simulink model "gimbal_cmd_unit_test"  (R2015b)
settings: Solver=FixedStepDiscrete  StartTime=0.0  StopTime=200  FixedStep=0.1  RelTol=1e-3
values from neighbouring files (symbols this model uses):
  Bm = 0.1    [gimbal_cmd_test.m]    (also in resolve_gimbal_angle_from_true_actuator_length.m)
  Jm = 0.01    [gimbal_cmd_test.m]    (also in resolve_gimbal_angle_from_true_actuator_length.m)
  Ke = 0.01    [gimbal_cmd_test.m]    (also in resolve_gimbal_angle_from_true_actuator_length.m)
  Kl = 500    [gimbal_cmd_test.m]    (also in resolve_gimbal_angle_from_true_actuator_length.m = 5000)
  Kt = 0.01    [gimbal_cmd_test.m]    (also in resolve_gimbal_angle_from_true_actuator_length.m)
  Lm = 0.5    [gimbal_cmd_test.m]    (also in resolve_gimbal_angle_from_true_actuator_length.m)
  mass = 50    [gimbal_cmd_test.m]
  nb = 2e-2/(2*pi)    (= 0.00318309886184)    [gimbal_cmd_test.m]    (also in resolve_gimbal_angle_from_true_actuator_length.m)
  Rm = 1    [gimbal_cmd_test.m]    (also in resolve_gimbal_angle_from_true_actuator_length.m)
  rot_err_x_rad = -1*pi/180    (= -0.0174532925199)    [gimbal_cmd_test.m]
  rot_err_y_rad = 0.0    (= 0)    [gimbal_cmd_test.m]
  rot_err_z_rad = 1*pi/180    (= 0.0174532925199)    [gimbal_cmd_test.m]
  w_err_x_rad = 0.0    (= 0)    [gimbal_cmd_test.m]
  w_err_y_rad = 0.0    (= 0)    [gimbal_cmd_test.m]
  w_err_z_rad = 0.0    (= 0)    [gimbal_cmd_test.m]
undefined symbols (not defined in the file or in its folder): DiscIntNeverNeededParam, tpl_x_gimbal_actuator_to_angle
libraries: util_quat_lib x2, simulink x1, simulink_extras x1, csc_vac_gimbal_steering_vernier_roll_acs_ctrl_lib_diag x1
settings Model: Creator=jimkaidy  LastModifiedBy=jimkaidy

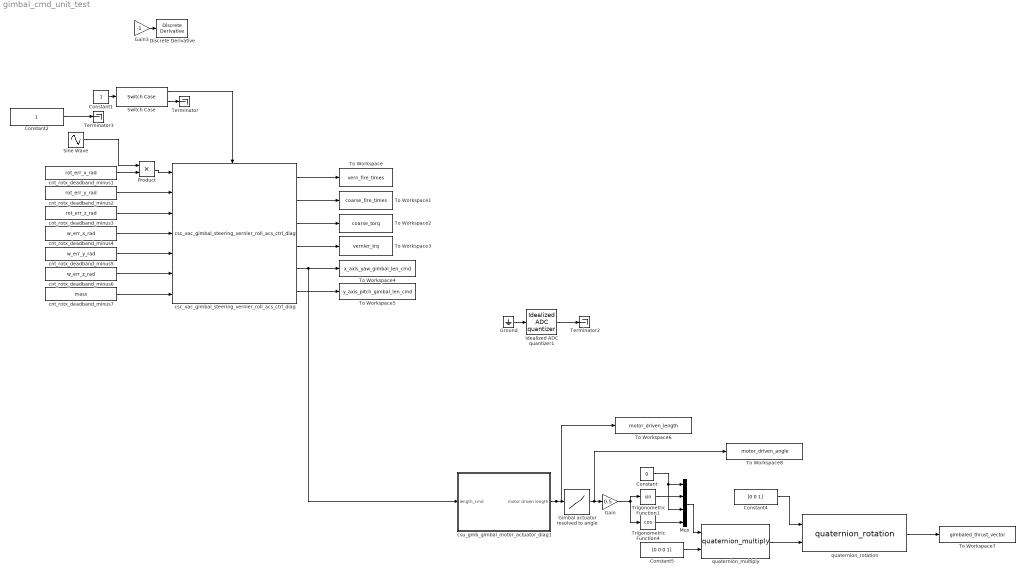
== system gimbal_cmd_unit_test ==
  Constant : Constant  Value=0
  Constant1 : Constant  OutDataTypeStr=uint8
  Constant2 : Constant  OutDataTypeStr=uint8
  Constant4 : Constant  Value=[0 0 1]
  Constant5 : Constant  Value=[0 0 0 1]
  Discrete Derivative : simulink/Discrete/Discrete Derivative  gainval=1.0  ICPrevScaledInput=0.0  InputProcessing=Inherited  OutMin=[]  OutMax=[]  OutDataType=fixdt(1, 16)  OutScaling=2^-10  DoSatur=off
  Gain : Gain  Gain=0.5
  Gain3 : Gain  Gain=-1
  Gimbal actuator resolved to angle : Lookup  InputValues=tpl_x_gimbal_actuator_to_angle(:,1)  Table=tpl_x_gimbal_actuator_to_angle(:,2)  LookUpMeth=Interpolation-Use End Values
  Ground : Ground
  Idealized ADC quantizer1 : simulink_extras/Additional Discrete/Idealized ADC quantizer  NumberOfConverterBits=12  Vmin=-10  Vmax=10  OutputDataType=int16  OutputNegativeValues=off
  Mux : Mux
  Product : Product
  Sine Wave : Sin  Frequency=10*pi/180  SampleTime=0.1
  Switch Case : SwitchCase
  Terminator : Terminator
  Terminator2 : Terminator
  Terminator3 : Terminator
  To Workspace : ToWorkspace  VariableName=vern_fire_times  SaveFormat=Timeseries  SampleTime=-1
  To Workspace1 : ToWorkspace  VariableName=coarse_fire_times  SaveFormat=Timeseries  SampleTime=-1
  To Workspace2 : ToWorkspace  VariableName=coarse_torq  SaveFormat=Timeseries  SampleTime=-1
  To Workspace3 : ToWorkspace  VariableName=vernier_trq  SaveFormat=Timeseries  SampleTime=-1
  To Workspace4 : ToWorkspace  VariableName=x_axis_yaw_gimbal_len_cmd  SaveFormat=Timeseries  SampleTime=-1
  To Workspace5 : ToWorkspace  VariableName=y_axis_pitch_gimbal_len_cmd  SaveFormat=Timeseries  SampleTime=-1
  To Workspace6 : ToWorkspace  VariableName=motor_driven_length  SaveFormat=Timeseries  SampleTime=-1
  To Workspace7 : ToWorkspace  VariableName=gimbaled_thrust_vector  SaveFormat=Timeseries  SampleTime=-1
  To Workspace8 : ToWorkspace  VariableName=motor_driven_angle  SaveFormat=Timeseries  SampleTime=-1
  Trigonometric Function1 : Trigonometry
  Trigonometric Function4 : Trigonometry  Operator=cos
  cnt_rotx_deadband_minus1 : Constant  Value=rot_err_x_rad
  cnt_rotx_deadband_minus2 : Constant  Value=rot_err_y_rad
  cnt_rotx_deadband_minus3 : Constant  Value=rot_err_z_rad
  cnt_rotx_deadband_minus4 : Constant  Value=w_err_x_rad
  cnt_rotx_deadband_minus5 : Constant  Value=w_err_y_rad
  cnt_rotx_deadband_minus6 : Constant  Value=w_err_z_rad
  cnt_rotx_deadband_minus7 : Constant  Value=mass
  csc_vac_gimbal_steering_vernier_roll_acs_ctrl_diag : csc_vac_gimbal_steering_vernier_roll_acs_ctrl_lib_diag/csc_vac_gimbal_steering_vernier_roll_acs_ctrl_diag
  csu_gmb_gimbal_motor_actuator_diag1 : Subsystem
  quaternion_multiply : util_quat_lib/quaternion_multiply  SystemSampleTime=-1
  quaternion_rotation : util_quat_lib/quaternion_rotation  SystemSampleTime=-1
  wires:
  cnt_rotx_deadband_minus7/1 -> csc_vac_gimbal_steering_vernier_roll_acs_ctrl_diag/7
  cnt_rotx_deadband_minus2/1 -> csc_vac_gimbal_steering_vernier_roll_acs_ctrl_diag/2
  cnt_rotx_deadband_minus3/1 -> csc_vac_gimbal_steering_vernier_roll_acs_ctrl_diag/3
  cnt_rotx_deadband_minus5/1 -> csc_vac_gimbal_steering_vernier_roll_acs_ctrl_diag/5
  cnt_rotx_deadband_minus6/1 -> csc_vac_gimbal_steering_vernier_roll_acs_ctrl_diag/6
  csc_vac_gimbal_steering_vernier_roll_acs_ctrl_diag/1 -> To Workspace/1
  csc_vac_gimbal_steering_vernier_roll_acs_ctrl_diag/2 -> To Workspace1/1
  csc_vac_gimbal_steering_vernier_roll_acs_ctrl_diag/3 -> To Workspace2/1
  csc_vac_gimbal_steering_vernier_roll_acs_ctrl_diag/4 -> To Workspace3/1
  csc_vac_gimbal_steering_vernier_roll_acs_ctrl_diag/6 -> To Workspace5/1
  Constant1/1 -> Switch Case/1
  Switch Case/1 -> csc_vac_gimbal_steering_vernier_roll_acs_ctrl_diag/Action
  Switch Case/2 -> Terminator/1
  Product/1 -> csc_vac_gimbal_steering_vernier_roll_acs_ctrl_diag/1
  cnt_rotx_deadband_minus1/1 -> Product/2
  Sine Wave/1 -> Product/1
  cnt_rotx_deadband_minus4/1 -> csc_vac_gimbal_steering_vernier_roll_acs_ctrl_diag/4
  Idealized ADC quantizer1/1 -> Terminator2/1
  Ground/1 -> Idealized ADC quantizer1/1
  csu_gmb_gimbal_motor_actuator_diag1/1(motor driven length) -> To Workspace6/1, Gimbal actuator resolved to angle/1
  Gimbal actuator resolved to angle/1 -> To Workspace8/1, Gain/1
  Gain/1 -> Trigonometric Function4/1, Trigonometric Function1/1
  Trigonometric Function4/1 -> Mux/4
  Trigonometric Function1/1 -> Mux/2
  Constant/1 -> Mux/3, Mux/1
  Mux/1 -> quaternion_multiply/1
  quaternion_multiply/1 -> quaternion_rotation/2
  Constant4/1 -> quaternion_rotation/1
  quaternion_rotation/1 -> To Workspace7/1
  csc_vac_gimbal_steering_vernier_roll_acs_ctrl_diag/5 -> csu_gmb_gimbal_motor_actuator_diag1/1(length_cmd), To Workspace4/1
  Constant5/1 -> quaternion_multiply/2
  Gain3/1 -> Discrete Derivative/1
  Constant2/1 -> Terminator3/1

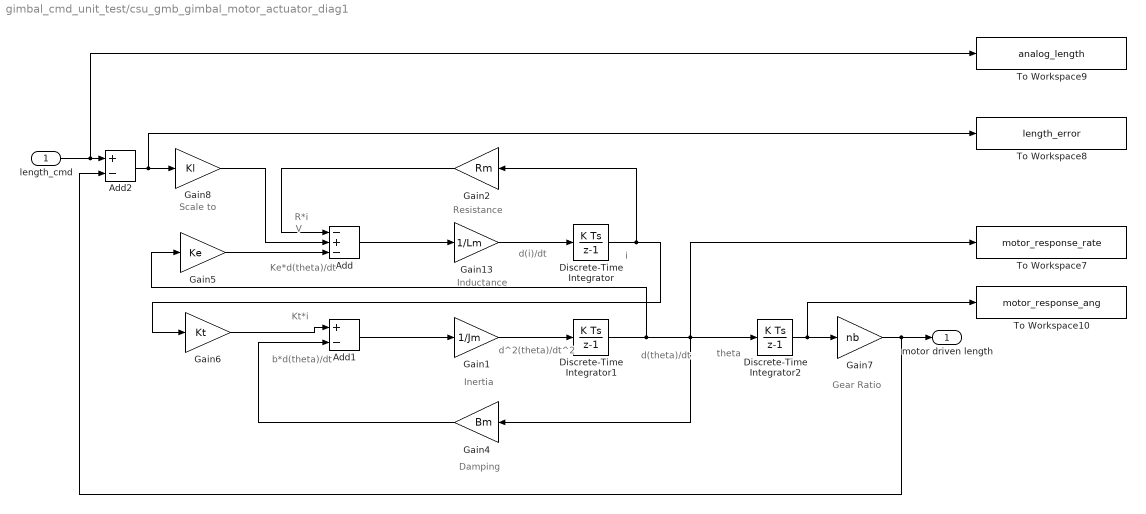
== system gimbal_cmd_unit_test/csu_gmb_gimbal_motor_actuator_diag1 ==
  note: Scale to
  note: theta
  note: d^2(theta)/dt^2
  note: b*d(theta)/dt
  note: Kt*i
  note: d(theta)/dt
  note: Ke*d(theta)/dt
  note: V
  note: R*i
  note: i
  note: d(i)/dt
  note: Gear Ratio
  note: Resistance
  note: Damping
  note: Inertia
  note: Inductance
  length_cmd : Inport
  Add : Sum  Inputs=-+-
  Add1 : Sum  Inputs=+-
  Add2 : Sum  Inputs=+-
  Discrete-Time Integrator : DiscreteIntegrator  InitialConditionSetting=State (most efficient)  SampleTime=-1  ICPrevOutput=DiscIntNeverNeededParam  ICPrevScaledInput=DiscIntNeverNeededParam
  Discrete-Time Integrator1 : DiscreteIntegrator  InitialConditionSetting=State (most efficient)  SampleTime=-1  ICPrevOutput=DiscIntNeverNeededParam  ICPrevScaledInput=DiscIntNeverNeededParam
  Discrete-Time Integrator2 : DiscreteIntegrator  InitialConditionSetting=State (most efficient)  SampleTime=-1  ICPrevOutput=DiscIntNeverNeededParam  ICPrevScaledInput=DiscIntNeverNeededParam
  Gain1 : Gain  Gain=1/Jm
  Gain13 : Gain  Gain=1/Lm
  Gain2 : Gain  Gain=Rm
  Gain4 : Gain  Gain=Bm
  Gain5 : Gain  Gain=Ke
  Gain6 : Gain  Gain=Kt
  Gain7 : Gain  Gain=nb
  Gain8 : Gain  Gain=Kl
  To Workspace10 : ToWorkspace  VariableName=motor_response_ang  SaveFormat=Timeseries  SampleTime=-1
  To Workspace7 : ToWorkspace  VariableName=motor_response_rate  SaveFormat=Timeseries  SampleTime=-1
  To Workspace8 : ToWorkspace  VariableName=length_error  SaveFormat=Timeseries  SampleTime=-1
  To Workspace9 : ToWorkspace  VariableName=analog_length  SaveFormat=Timeseries  SampleTime=-1
  motor driven length : Outport
  wires:
  length_cmd/1 -> To Workspace9/1, Add2/1
  Gain13/1 -> Discrete-Time Integrator/1
  Gain1/1 -> Discrete-Time Integrator1/1
  Gain5/1 -> Add/3
  Gain4/1 -> Add1/2
  Gain2/1 -> Add/1
  Gain6/1 -> Add1/1
  Discrete-Time Integrator/1 -> Gain2/1, Gain6/1
  Gain8/1 -> Add/2
  Add/1 -> Gain13/1
  Add1/1 -> Gain1/1
  Discrete-Time Integrator1/1 -> Gain5/1, To Workspace7/1, Gain4/1, Discrete-Time Integrator2/1
  Add2/1 -> To Workspace8/1, Gain8/1
  Discrete-Time Integrator2/1 -> To Workspace10/1, Gain7/1
  Gain7/1 -> Add2/2, motor driven length/1
